simulink model "torqueBalancingSOT2012b"  (Simulink 8.0)
settings: Solver=FixedStepDiscrete  StartTime=0.0  StopTime=CONFIG.SIMULATION_TIME  FixedStep=CONFIG.Ts  RelTol=1e-3
InitFcn:
  | cd(fileparts(which(bdroot)));
  | initTorqueBalancingSOT;
undefined symbols (not defined in the file or in its folder): CONFIG, ConstraintsFeetMatrix, gain, ROBOT_DOF, sat, sm, upperBoundFeetConstraints, WBT_robotName
libraries: WBToolboxLibrary x51
(part 1 of 2)
settings Model: Creator=marie  LastModifiedBy=marie  CovMetricSettings=dwe  CovHtmlReporting=off  covSaveCumulativeToWorkspaceVar=off  CovSaveSingleToWorkspaceVar=off  CovExternalEMLEnable=on
settings DataIOCC: LimitDataPoints=off  SaveFormat=StructureWithTime
settings OptimizationCC: ExpressionDepthLimit=128
settings DebuggingCC: UnderspecifiedInitializationDetection=Simplified  MergeDetectMultiDrivingBlocksExec=error  SolverPrmCheckMsg=none  FrameProcessingCompatibilityMsg=error  StateNameClashWarn=none  SFUnexpectedBacktrackingDiag=error  SFNoUnconditionalDefaultTransitionDiag=error
settings HardwareCC: ProdBitPerPointer=64  ProdLargestAtomicFloat=Float  ProdIntDivRoundTo=Zero  ProdEndianess=LittleEndian  ProdHWDeviceType=Specified
settings ModelReferenceCC: PropagateSignalLabelsOutOfModel=on
settings CodeAppCC: CustomSymbolStrType=$N$R$M_T
settings GRTTargetCC: CodeReplacementLibrary=C99 (ISO)  GeneratePreprocessorConditionals=Use local settings

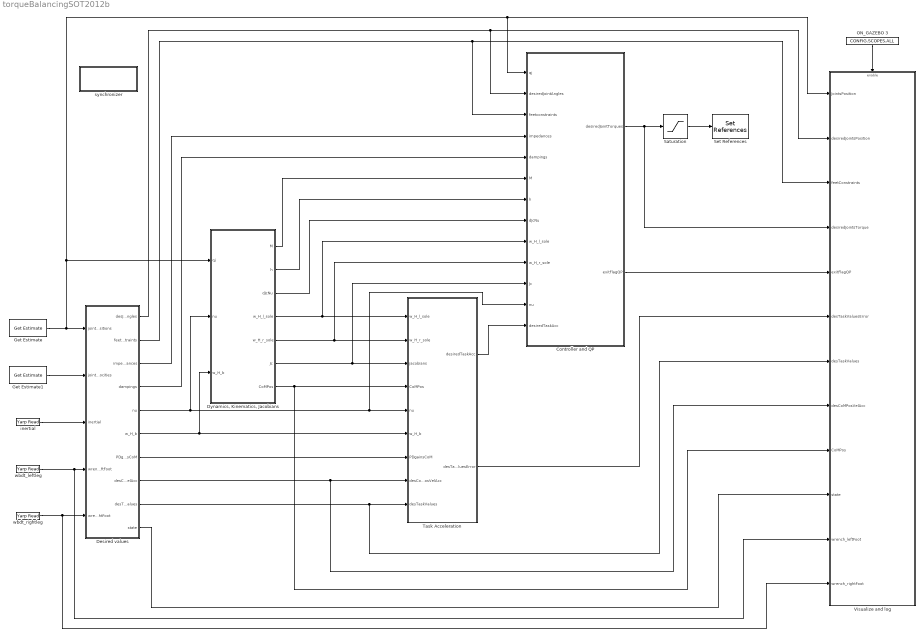
== system torqueBalancingSOT2012b ==
  Controller and QP : Subsystem
  Desired values : Subsystem
  "Dynamics, Kinematics, Jacobians" : Subsystem
  Get Estimate : WBToolboxLibrary/wholeBodyStates/Get Estimate  estimateType=Joints Position  robotName=WBT_robotName  localName=WBT_modelName  wbiFile=WBT_wbiFilename  wbiList=WBT_wbiList
  Get Estimate1 : WBToolboxLibrary/wholeBodyStates/Get Estimate  estimateType=Joints Velocity  robotName=WBT_robotName  localName=WBT_modelName  wbiFile=WBT_wbiFilename  wbiList=WBT_wbiList
  ON_GAZEBO 3 : Constant  Value=CONFIG.SCOPES.ALL
  Saturation : Saturate  UpperLimit=sat.torque  LowerLimit=-sat.torque
  Set References : WBToolboxLibrary/wholeBodyActuators/Set References  controlType=Torque  fullOrSubControl=Full  controlledJoints=''  robotName=WBT_robotName  localName=WBT_modelName  wbiFile=WBT_wbiFilename  wbiList=WBT_wbiList
  Task Acceleration : Subsystem
  Visualize and log : Subsystem
  inertial : WBToolboxLibrary/Utilities/Yarp Read  portName=PORTS.IMU  signalSize=12  blocking=off  timestamp=off  autoconnect=on  errorOnConnection=on
  synchronizer : Subsystem
      mask Display: disp('SYNCHRONIZER')
  wbdt_leftleg : WBToolboxLibrary/Utilities/Yarp Read  portName=PORTS.WBDT_LEFTLEG_EE  signalSize=6  blocking=off  timestamp=off  autoconnect=on  errorOnConnection=off
  wbdt_rightleg : WBToolboxLibrary/Utilities/Yarp Read  portName=PORTS.WBDT_RIGHTLEG_EE  signalSize=6  blocking=off  timestamp=off  autoconnect=on  errorOnConnection=off
  wires:
  Desired values/6(w_H_b) -> Task Acceleration/6(w_H_b), "Dynamics, Kinematics, Jacobians"/3(w_H_b)
  Get Estimate/1 -> "Dynamics, Kinematics, Jacobians"/1(qj), Visualize and log/1(JointsPosition), Controller and QP/1(qj), Desired values/1(jointPositions)
  "Dynamics, Kinematics, Jacobians"/7(CoMPos) -> Visualize and log/9(CoMPos), Task Acceleration/4(CoMPos)
  Desired values/8(desCoMPosVelAcc) -> Visualize and log/8(desCoMPosVelAcc), Task Acceleration/8(desCoMPosVelAcc)
  Desired values/5(nu) -> Controller and QP/12(nu), Task Acceleration/5(nu), "Dynamics, Kinematics, Jacobians"/2(nu)
  "Dynamics, Kinematics, Jacobians"/6(Jc) -> Controller and QP/11(Jc), Task Acceleration/3(jacobians)
  Desired values/1(desJointAngles) -> Controller and QP/2(desiredJointAngles), Visualize and log/2(desiredJointsPosition)
  Desired values/9(desTaskValues) -> Task Acceleration/9(desTaskValues), Visualize and log/7(desTaskValues)
  Desired values/7(PDgainsCoM) -> Task Acceleration/7(PDgainsCoM)
  "Dynamics, Kinematics, Jacobians"/5(w_H_r_sole) -> Controller and QP/10(w_H_r_sole), Task Acceleration/2(w_H_r_sole)
  "Dynamics, Kinematics, Jacobians"/4(w_H_l_sole) -> Controller and QP/9(w_H_l_sole), Task Acceleration/1(w_H_l_sole)
  Desired values/3(impedances) -> Controller and QP/4(impedances)
  Desired values/2(feetConstraints) -> Visualize and log/3(feetConstraints), Controller and QP/3(feetconstraints)
  "Dynamics, Kinematics, Jacobians"/1(M) -> Controller and QP/6(M)
  "Dynamics, Kinematics, Jacobians"/2(h) -> Controller and QP/7(h)
  "Dynamics, Kinematics, Jacobians"/3(dJcNu) -> Controller and QP/8(dJcNu)
  Task Acceleration/1(desiredTaskAcc) -> Controller and QP/13(desiredTaskAcc)
  Desired values/4(dampings) -> Controller and QP/5(dampings)
  Controller and QP/1(desiredJointTorques) -> Visualize and log/4(desiredJointsTorque), Saturation/1
  Saturation/1 -> Set References/1
  ON_GAZEBO 3/1 -> Visualize and log/Enable
  Desired values/10(state) -> Visualize and log/10(state)
  Controller and QP/2(exitFlagQP) -> Visualize and log/5(exitFlagQP)
  Task Acceleration/2(desTaskValuesError) -> Visualize and log/6(desTaskValuesError)
  inertial/1 -> Desired values/3(inertial)
  wbdt_leftleg/1 -> Desired values/4(wrench_leftFoot), Visualize and log/11(wrench_leftFoot)
  wbdt_rightleg/1 -> Desired values/5(wrench_rightFoot), Visualize and log/12(wrench_rightFoot)
  Get Estimate1/1 -> Desired values/2(jointVelocities)

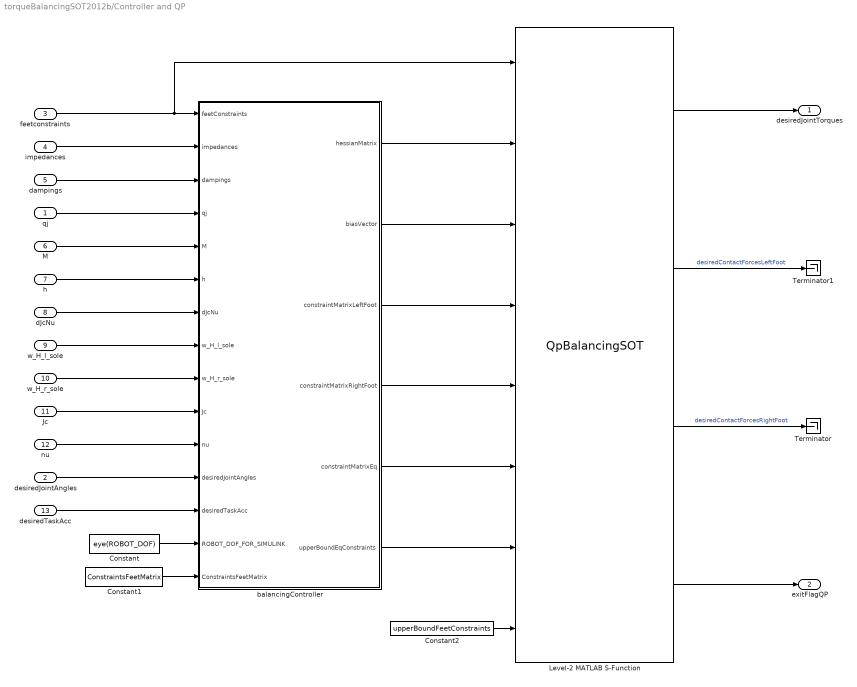
== system torqueBalancingSOT2012b/Controller and QP ==
  qj : Inport
  desiredJointAngles : Inport  Port=2
  feetconstraints : Inport  Port=3
  impedances : Inport  Port=4
  dampings : Inport  Port=5
  M : Inport  Port=6
  h : Inport  Port=7
  dJcNu : Inport  Port=8
  w_H_l_sole : Inport  Port=9
  w_H_r_sole : Inport  Port=10
  Jc : Inport  Port=11
  nu : Inport  Port=12
  desiredTaskAcc : Inport  Port=13
  Constant : Constant  Value=eye(ROBOT_DOF)
  Constant1 : Constant  Value=ConstraintsFeetMatrix
  Constant2 : Constant  Value=upperBoundFeetConstraints
  Level-2 MATLAB S-Function : M-S-Function  FunctionName=QpBalancingSOT  Parameters=ROBOT_DOF,sat.torqueDot,CONFIG.Ts,CONFIG.QP.USE_CONTINUITY_CONSTRAINTS,CONFIG.QP.USE_STRICT_TASK_PRIORITIES, reg.HessianQP  mask{robotDofs=ROBOT_DOF, tauDotMax=sat.torqueDot, Ts=CONFIG.Ts}
      mask prompts: robotDofs "Robt degrees of freedom"; tauDotMax "Maximum derivative of torques"; Ts "Controller period"
      mask Display: disp('QP')
  Terminator : Terminator
  Terminator1 : Terminator
  balancingController : MATLAB Function  TreatAsAtomicUnit=on
      settings: PermitHierarchicalResolution=ParametersOnly
  desiredJointTorques : Outport
  exitFlagQP : Outport  Port=2
  wires:
  balancingController/1(hessianMatrix) -> Level-2 MATLAB S-Function/2
  feetconstraints/1 -> balancingController/1(feetConstraints), Level-2 MATLAB S-Function/1
  qj/1 -> balancingController/4(qj)
  impedances/1 -> balancingController/2(impedances)
  M/1 -> balancingController/5(M)
  h/1 -> balancingController/6(h)
  dJcNu/1 -> balancingController/7(dJcNu)
  w_H_l_sole/1 -> balancingController/8(w_H_l_sole)
  w_H_r_sole/1 -> balancingController/9(w_H_r_sole)
  Jc/1 -> balancingController/10(Jc)
  nu/1 -> balancingController/11(nu)
  desiredJointAngles/1 -> balancingController/12(desiredJointAngles)
  desiredTaskAcc/1 -> balancingController/13(desiredTaskAcc)
  Constant/1 -> balancingController/14(ROBOT_DOF_FOR_SIMULINK)
  Constant1/1 -> balancingController/15(ConstraintsFeetMatrix)
  dampings/1 -> balancingController/3(dampings)
  balancingController/2(biasVector) -> Level-2 MATLAB S-Function/3
  balancingController/3(constraintMatrixLeftFoot) -> Level-2 MATLAB S-Function/4
  balancingController/4(constraintMatrixRightFoot) -> Level-2 MATLAB S-Function/5
  balancingController/5(constraintMatrixEq) -> Level-2 MATLAB S-Function/6
  balancingController/6(upperBoundEqConstraints) -> Level-2 MATLAB S-Function/7
  Constant2/1 -> Level-2 MATLAB S-Function/8
  Level-2 MATLAB S-Function/1 -> desiredJointTorques/1
  Level-2 MATLAB S-Function/2 -> Terminator1/1  "desiredContactForcesLeftFoot"
  Level-2 MATLAB S-Function/3 -> Terminator/1  "desiredContactForcesRightFoot"
  Level-2 MATLAB S-Function/4 -> exitFlagQP/1

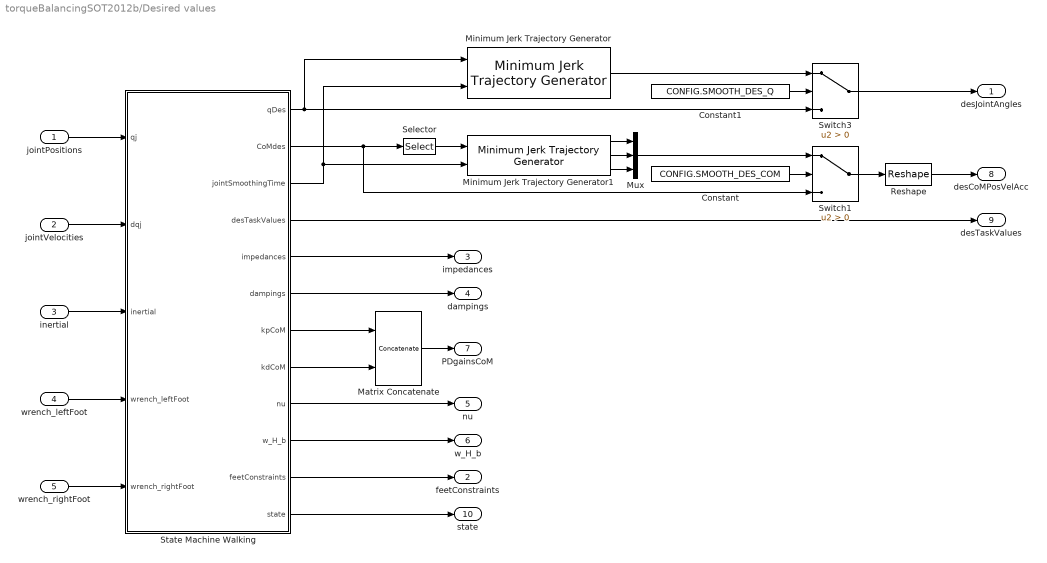
== system torqueBalancingSOT2012b/Desired values ==
  jointPositions : Inport
  jointVelocities : Inport  Port=2
  inertial : Inport  Port=3
  wrench_leftFoot : Inport  Port=4
  wrench_rightFoot : Inport  Port=5
  Constant : Constant  Value=CONFIG.SMOOTH_DES_COM
  Constant1 : Constant  Value=CONFIG.SMOOTH_DES_Q
  Matrix Concatenate : Concatenate  Mode=Multidimensional array  ConcatenateDimension=2
  Minimum Jerk Trajectory Generator : WBToolboxLibrary/Utilities/Minimum Jerk Trajectory Generator  externalSettlingTime=on  settlingTime=3  sampleTime=CONFIG.Ts  resetOnSettlingTime=off  firstDerivatives=off  secondDerivatives=off  explicitInitialValue=off
  Minimum Jerk Trajectory Generator1 : WBToolboxLibrary/Utilities/Minimum Jerk Trajectory Generator  externalSettlingTime=on  settlingTime=3  sampleTime=CONFIG.Ts  resetOnSettlingTime=off  firstDerivatives=on  secondDerivatives=on  explicitInitialValue=off
  Mux : Mux  Inputs=3
  Reshape : Reshape  OutputDimensionality=Customize  OutputDimensions=[3,3]
  Selector : Selector  InputPortWidth=9  IndexOptions=Index vector (dialog)  Indices=[1 2 3]  OutputSizes=1
  State Machine Walking : Subsystem
  Switch1 : Switch  Criteria=u2 > Threshold
  Switch3 : Switch  Criteria=u2 > Threshold
  desJointAngles : Outport
  feetConstraints : Outport  Port=2
  impedances : Outport  Port=3
  dampings : Outport  Port=4
  nu : Outport  Port=5
  w_H_b : Outport  Port=6
  PDgainsCoM : Outport  Port=7
  desCoMPosVelAcc : Outport  Port=8
  desTaskValues : Outport  Port=9
  state : Outport  Port=10
  wires:
  Minimum Jerk Trajectory Generator/1 -> Switch3/1
  Constant/1 -> Switch1/2
  Constant1/1 -> Switch3/2
  Minimum Jerk Trajectory Generator1/3 -> Mux/3
  Minimum Jerk Trajectory Generator1/2 -> Mux/2
  State Machine Walking/8(kdCoM) -> Matrix Concatenate/2
  Matrix Concatenate/1 -> PDgainsCoM/1
  State Machine Walking/10(w_H_b) -> w_H_b/1
  State Machine Walking/12(state) -> state/1
  Mux/1 -> Switch1/1
  Minimum Jerk Trajectory Generator1/1 -> Mux/1
  State Machine Walking/5(impedances) -> impedances/1
  Selector/1 -> Minimum Jerk Trajectory Generator1/1
  State Machine Walking/3(jointSmoothingTime) -> Minimum Jerk Trajectory Generator/2, Minimum Jerk Trajectory Generator1/2
  Switch1/1 -> Reshape/1
  Switch3/1 -> desJointAngles/1
  State Machine Walking/2(CoMdes) -> Switch1/3, Selector/1
  State Machine Walking/4(desTaskValues) -> desTaskValues/1
  State Machine Walking/11(feetConstraints) -> feetConstraints/1
  State Machine Walking/1(qDes) -> Minimum Jerk Trajectory Generator/1, Switch3/3
  State Machine Walking/9(nu) -> nu/1
  State Machine Walking/7(kpCoM) -> Matrix Concatenate/1
  Reshape/1 -> desCoMPosVelAcc/1
  jointPositions/1 -> State Machine Walking/1(qj)
  jointVelocities/1 -> State Machine Walking/2(dqj)
  State Machine Walking/6(dampings) -> dampings/1
  wrench_rightFoot/1 -> State Machine Walking/5(wrench_rightFoot)
  wrench_leftFoot/1 -> State Machine Walking/4(wrench_leftFoot)
  inertial/1 -> State Machine Walking/3(inertial)

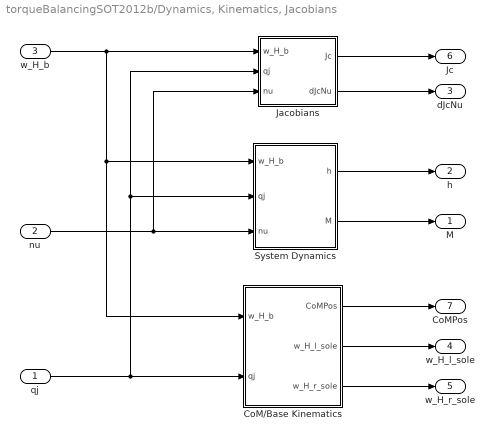
== system torqueBalancingSOT2012b/Dynamics, Kinematics, Jacobians ==
  qj : Inport
  nu : Inport  Port=2
  w_H_b : Inport  Port=3
  CoM/Base Kinematics : Subsystem
  Jacobians : Subsystem
  System Dynamics : Subsystem
  M : Outport
  h : Outport  Port=2
  dJcNu : Outport  Port=3
  w_H_l_sole : Outport  Port=4
  w_H_r_sole : Outport  Port=5
  Jc : Outport  Port=6
  CoMPos : Outport  Port=7
  wires:
  qj/1 -> Jacobians/2(qj), System Dynamics/2(qj), CoM/Base Kinematics/2(qj)
  w_H_b/1 -> CoM/Base Kinematics/1(w_H_b), System Dynamics/1(w_H_b), Jacobians/1(w_H_b)
  CoM/Base Kinematics/1(CoMPos) -> CoMPos/1
  nu/1 -> Jacobians/3(nu), System Dynamics/3(nu)
  Jacobians/1(Jc) -> Jc/1
  Jacobians/2(dJcNu) -> dJcNu/1
  System Dynamics/2(M) -> M/1
  System Dynamics/1(h) -> h/1
  CoM/Base Kinematics/2(w_H_l_sole) -> w_H_l_sole/1
  CoM/Base Kinematics/3(w_H_r_sole) -> w_H_r_sole/1

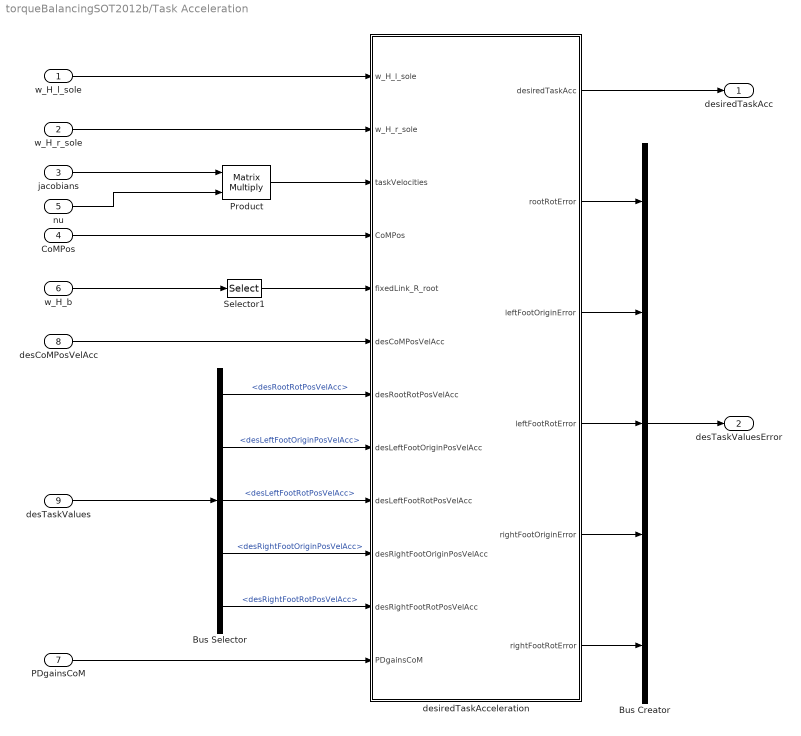
== system torqueBalancingSOT2012b/Task Acceleration ==
  w_H_l_sole : Inport
  w_H_r_sole : Inport  Port=2
  jacobians : Inport  Port=3
  CoMPos : Inport  Port=4
  nu : Inport  Port=5
  w_H_b : Inport  Port=6
  PDgainsCoM : Inport  Port=7
  desCoMPosVelAcc : Inport  Port=8
  desTaskValues : Inport  Port=9
  Bus Creator : BusCreator  Inputs='rootRotError','leftFootOriginError','leftFootRotError','rightFootOriginError','rightFootRotError'
  Bus Selector : BusSelector  OutputSignals=desRootRotPosVelAcc,desLeftFootOriginPosVelAcc,desLeftFootRotPosVelAcc,desRightFootOriginPosVelAcc,desRightFootRotPosVelAcc
  Product : Product  Multiplication=Matrix(*)
  Selector1 : Selector  NumberOfDimensions=2  InputPortWidth=9  IndexOptions=Index vector (dialog),Index vector (dialog)  Indices=[1:3],[1:3]  OutputSizes=1,1
  desiredTaskAcceleration : MATLAB Function  TreatAsAtomicUnit=on
      settings: PermitHierarchicalResolution=ParametersOnly
  desiredTaskAcc : Outport
  desTaskValuesError : Outport  Port=2
  wires:
  Bus Selector/1 -> desiredTaskAcceleration/7(desRootRotPosVelAcc)  "<desRootRotPosVelAcc>"
  Bus Selector/2 -> desiredTaskAcceleration/8(desLeftFootOriginPosVelAcc)  "<desLeftFootOriginPosVelAcc>"
  Bus Selector/3 -> desiredTaskAcceleration/9(desLeftFootRotPosVelAcc)  "<desLeftFootRotPosVelAcc>"
  Bus Selector/4 -> desiredTaskAcceleration/10(desRightFootOriginPosVelAcc)  "<desRightFootOriginPosVelAcc>"
  desTaskValues/1 -> Bus Selector/1
  w_H_b/1 -> Selector1/1
  Bus Selector/5 -> desiredTaskAcceleration/11(desRightFootRotPosVelAcc)  "<desRightFootRotPosVelAcc>"
  PDgainsCoM/1 -> desiredTaskAcceleration/12(PDgainsCoM)
  jacobians/1 -> Product/1
  nu/1 -> Product/2
  CoMPos/1 -> desiredTaskAcceleration/4(CoMPos)
  desCoMPosVelAcc/1 -> desiredTaskAcceleration/6(desCoMPosVelAcc)
  Product/1 -> desiredTaskAcceleration/3(taskVelocities)
  desiredTaskAcceleration/2(rootRotError) -> Bus Creator/1
  desiredTaskAcceleration/3(leftFootOriginError) -> Bus Creator/2
  desiredTaskAcceleration/4(leftFootRotError) -> Bus Creator/3
  desiredTaskAcceleration/5(rightFootOriginError) -> Bus Creator/4
  desiredTaskAcceleration/6(rightFootRotError) -> Bus Creator/5
  desiredTaskAcceleration/1(desiredTaskAcc) -> desiredTaskAcc/1
  Bus Creator/1 -> desTaskValuesError/1
  w_H_r_sole/1 -> desiredTaskAcceleration/2(w_H_r_sole)
  w_H_l_sole/1 -> desiredTaskAcceleration/1(w_H_l_sole)
  Selector1/1 -> desiredTaskAcceleration/5(fixedLink_R_root)

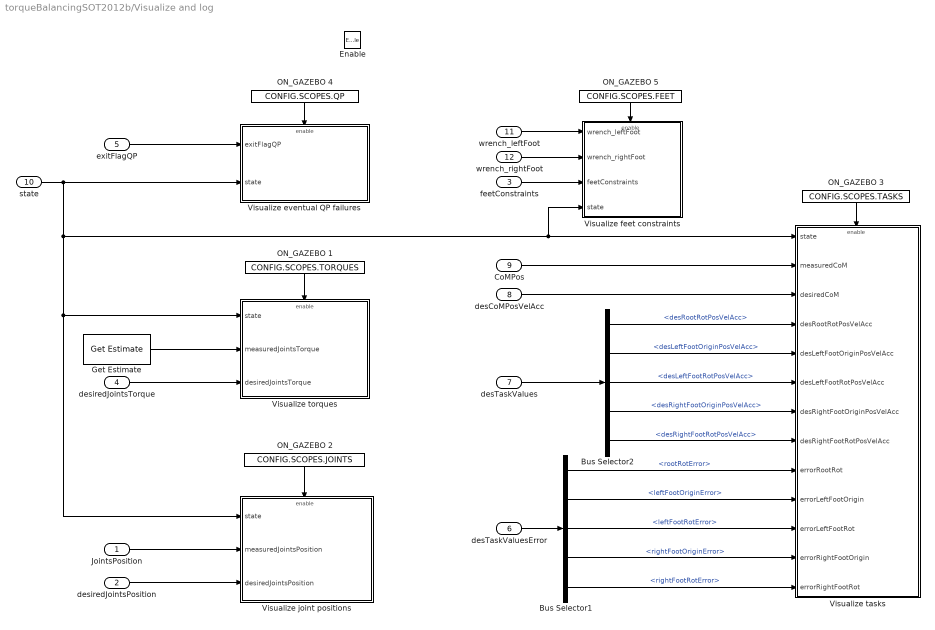
== system torqueBalancingSOT2012b/Visualize and log ==
  JointsPosition : Inport
  desiredJointsPosition : Inport  Port=2
  feetConstraints : Inport  Port=3
  desiredJointsTorque : Inport  Port=4
  exitFlagQP : Inport  Port=5
  desTaskValuesError : Inport  Port=6
  desTaskValues : Inport  Port=7
  desCoMPosVelAcc : Inport  Port=8
  CoMPos : Inport  Port=9
  state : Inport  Port=10
  wrench_leftFoot : Inport  Port=11
  wrench_rightFoot : Inport  Port=12
  Enable : EnablePort
  Bus Selector1 : BusSelector  OutputSignals=rootRotError,leftFootOriginError,leftFootRotError,rightFootOriginError,rightFootRotError
  Bus Selector2 : BusSelector  OutputSignals=desRootRotPosVelAcc,desLeftFootOriginPosVelAcc,desLeftFootRotPosVelAcc,desRightFootOriginPosVelAcc,desRightFootRotPosVelAcc
  Get Estimate : WBToolboxLibrary/wholeBodyStates/Get Estimate  estimateType=Joints Torque  robotName=WBT_robotName  localName=WBT_modelName  wbiFile=WBT_wbiFilename  wbiList=WBT_wbiList
  ON_GAZEBO 1 : Constant  Value=CONFIG.SCOPES.TORQUES
  ON_GAZEBO 2 : Constant  Value=CONFIG.SCOPES.JOINTS
  ON_GAZEBO 3 : Constant  Value=CONFIG.SCOPES.TASKS
  ON_GAZEBO 4 : Constant  Value=CONFIG.SCOPES.QP
  ON_GAZEBO 5 : Constant  Value=CONFIG.SCOPES.FEET
  Visualize eventual QP failures : Subsystem
  Visualize feet constraints : Subsystem
  Visualize joint positions : Subsystem
  Visualize tasks : Subsystem
  Visualize torques : Subsystem
  wires:
  ON_GAZEBO 4/1 -> Visualize eventual QP failures/Enable
  exitFlagQP/1 -> Visualize eventual QP failures/1(exitFlagQP)
  Get Estimate/1 -> Visualize torques/2(measuredJointsTorque)
  desiredJointsTorque/1 -> Visualize torques/3(desiredJointsTorque)
  ON_GAZEBO 1/1 -> Visualize torques/Enable
  state/1 -> Visualize eventual QP failures/2(state), Visualize joint positions/1(state), Visualize torques/1(state), Visualize feet constraints/4(state), Visualize tasks/1(state)
  JointsPosition/1 -> Visualize joint positions/2(measuredJointsPosition)
  desiredJointsPosition/1 -> Visualize joint positions/3(desiredJointsPosition)
  ON_GAZEBO 2/1 -> Visualize joint positions/Enable
  CoMPos/1 -> Visualize tasks/2(measuredCoM)
  desCoMPosVelAcc/1 -> Visualize tasks/3(desiredCoM)
  Bus Selector2/3 -> Visualize tasks/6(desLeftFootRotPosVelAcc)  "<desLeftFootRotPosVelAcc>"
  Bus Selector2/2 -> Visualize tasks/5(desLeftFootOriginPosVelAcc)  "<desLeftFootOriginPosVelAcc>"
  Bus Selector2/5 -> Visualize tasks/8(desRightFootRotPosVelAcc)  "<desRightFootRotPosVelAcc>"
  Bus Selector2/4 -> Visualize tasks/7(desRightFootOriginPosVelAcc)  "<desRightFootOriginPosVelAcc>"
  desTaskValues/1 -> Bus Selector2/1
  Bus Selector2/1 -> Visualize tasks/4(desRootRotPosVelAcc)  "<desRootRotPosVelAcc>"
  desTaskValuesError/1 -> Bus Selector1/1
  Bus Selector1/1 -> Visualize tasks/9(errorRootRot)  "<rootRotError>"
  Bus Selector1/2 -> Visualize tasks/10(errorLeftFootOrigin)  "<leftFootOriginError>"
  Bus Selector1/3 -> Visualize tasks/11(errorLeftFootRot)  "<leftFootRotError>"
  Bus Selector1/4 -> Visualize tasks/12(errorRightFootOrigin)  "<rightFootOriginError>"
  Bus Selector1/5 -> Visualize tasks/13(errorRightFootRot)  "<rightFootRotError>"
  ON_GAZEBO 3/1 -> Visualize tasks/Enable
  feetConstraints/1 -> Visualize feet constraints/3(feetConstraints)
  ON_GAZEBO 5/1 -> Visualize feet constraints/Enable
  wrench_rightFoot/1 -> Visualize feet constraints/2(wrench_rightFoot)
  wrench_leftFoot/1 -> Visualize feet constraints/1(wrench_leftFoot)

== system torqueBalancingSOT2012b/synchronizer ==
  GAZEBO_SYNCHRONIZER : Subsystem
  Logical Operator : Logic  Operator=NOT  AllPortsSameDT=off  OutDataTypeStr=boolean
  "ON_GAZEBO " : Constant  Value=CONFIG.ON_GAZEBO
  REAL_TIME_SYNC : Subsystem
  wires:
  Logical Operator/1 -> REAL_TIME_SYNC/Enable
  "ON_GAZEBO "/1 -> GAZEBO_SYNCHRONIZER/Enable, Logical Operator/1

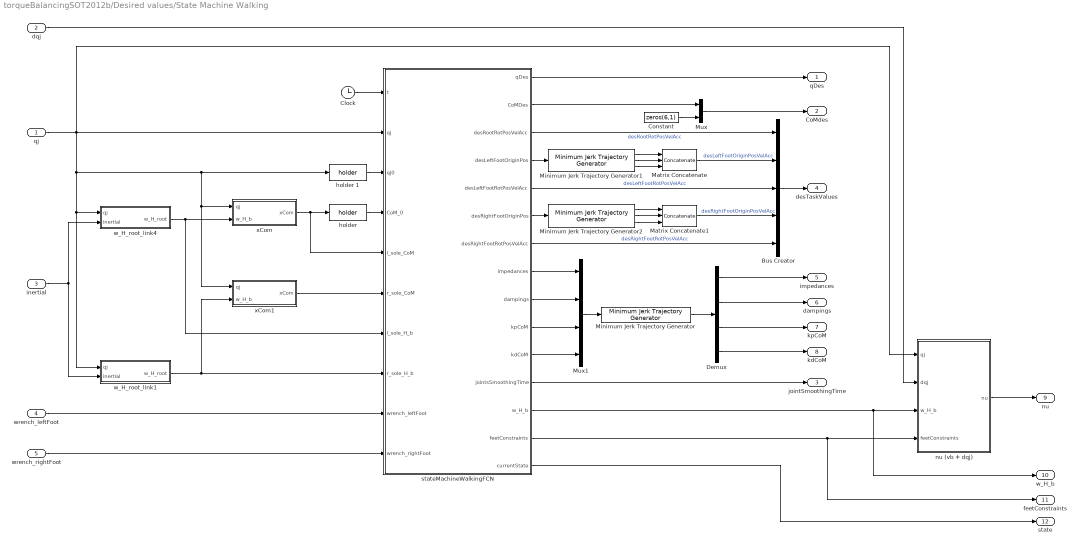
== system torqueBalancingSOT2012b/Desired values/State Machine Walking ==
  qj : Inport
  dqj : Inport  Port=2
  inertial : Inport  Port=3
  wrench_leftFoot : Inport  Port=4
  wrench_rightFoot : Inport  Port=5
  Bus Creator : BusCreator  Inputs='desRootRotPosVelAcc','desLeftFootOriginPosVelAcc','desLeftFootRotPosVelAcc','desRightFootOriginPosVelAcc','desRightFootRotPosVelAcc'
  Clock : Clock
  Constant : Constant  Value=zeros(6,1)
  Demux : Demux  Outputs=[ROBOT_DOF, ROBOT_DOF, 3, 3]
  Matrix Concatenate : Concatenate  NumInputs=3  Mode=Multidimensional array  ConcatenateDimension=2
  Matrix Concatenate1 : Concatenate  NumInputs=3  Mode=Multidimensional array  ConcatenateDimension=2
  Minimum Jerk Trajectory Generator : WBToolboxLibrary/Utilities/Minimum Jerk Trajectory Generator  externalSettlingTime=off  settlingTime=gain.SmoothingTimeGainScheduling  sampleTime=CONFIG.Ts  resetOnSettlingTime=off  firstDerivatives=off  secondDerivatives=off  explicitInitialValue=off
  Minimum Jerk Trajectory Generator1 : WBToolboxLibrary/Utilities/Minimum Jerk Trajectory Generator  externalSettlingTime=off  settlingTime=gain.SmoothingTimeGainScheduling  sampleTime=CONFIG.Ts  resetOnSettlingTime=off  firstDerivatives=on  secondDerivatives=on  explicitInitialValue=off
  Minimum Jerk Trajectory Generator2 : WBToolboxLibrary/Utilities/Minimum Jerk Trajectory Generator  externalSettlingTime=off  settlingTime=gain.SmoothingTimeGainScheduling  sampleTime=CONFIG.Ts  resetOnSettlingTime=off  firstDerivatives=on  secondDerivatives=on  explicitInitialValue=off
  Mux : Mux  Inputs=2
  Mux1 : Mux
  "holder " : WBToolboxLibrary/Utilities/holder 
  holder 1 : WBToolboxLibrary/Utilities/holder 
  nu (vb + dqj) : Subsystem
  stateMachineWalkingFCN : MATLAB Function  TreatAsAtomicUnit=on
      settings: PermitHierarchicalResolution=ParametersOnly
  w_H_root_link1 : Subsystem  mask{link_name='r_sole'}
      mask prompts: link_name "link name"
      mask help:
      | This block evaluates the homogeneous transformation between the world and the root link, i.e. ^wH_b. It assumes that the link specified by the variable 'link_name' has a constant position
      | w.r.t. an inertial frame, but it can rotate arbitrarily. This rotation is retrived from the IMU sensor.
      mask Display:
      | str = strrep(link_name, '_','\_');
      | port_label('output',1,['{}^{',str '}H_{root}'],'texmode','on')
      | clear str;
      | 
      | port_label('input',1,'q_j','texmode','on')
      | 
      | port_label('input',2,'inertial','texmode','on')
  w_H_root_link4 : Subsystem  mask{link_name='l_sole'}
      mask prompts: link_name "link name"
      mask help:
      | This block evaluates the homogeneous transformation between the world and the root link, i.e. ^wH_b. It assumes that the link specified by the variable 'link_name' has a constant position
      | w.r.t. an inertial frame, but it can rotate arbitrarily. This rotation is retrived from the IMU sensor.
      mask Display:
      | str = strrep(link_name, '_','\_');
      | port_label('output',1,['{}^{',str '}H_{root}'],'texmode','on')
      | clear str;
      | 
      | port_label('input',1,'q_j','texmode','on')
      | 
      | port_label('input',2,'inertial','texmode','on')
  xCom : Subsystem
  xCom1 : Subsystem
  qDes : Outport
  CoMdes : Outport  Port=2
  jointSmoothingTime : Outport  Port=3
  desTaskValues : Outport  Port=4
  impedances : Outport  Port=5
  dampings : Outport  Port=6
  kpCoM : Outport  Port=7
  kdCoM : Outport  Port=8
  nu : Outport  Port=9
  w_H_b : Outport  Port=10
  feetConstraints : Outport  Port=11
  state : Outport  Port=12
  wires:
  Clock/1 -> stateMachineWalkingFCN/1(t)
  stateMachineWalkingFCN/8(impedances) -> Mux1/1
  stateMachineWalkingFCN/11(kdCoM) -> Mux1/4
  stateMachineWalkingFCN/7(desRightFootRotPosVelAcc) -> Bus Creator/5  "desRightFootRotPosVelAcc"
  Bus Creator/1 -> desTaskValues/1
  wrench_rightFoot/1 -> stateMachineWalkingFCN/10(wrench_rightFoot)
  stateMachineWalkingFCN/10(kpCoM) -> Mux1/3
  stateMachineWalkingFCN/13(w_H_b) -> w_H_b/1, nu (vb + dqj)/3(w_H_b)
  wrench_leftFoot/1 -> stateMachineWalkingFCN/9(wrench_leftFoot)
  Mux1/1 -> Minimum Jerk Trajectory Generator/1
  qj/1 -> nu (vb + dqj)/1(qj), w_H_root_link1/1(qj), w_H_root_link4/1(qj), xCom1/1(qj), xCom/1(qj), holder 1/1, stateMachineWalkingFCN/2(qj)
  nu (vb + dqj)/1(nu) -> nu/1
  holder 1/1 -> stateMachineWalkingFCN/3(qj0)
  xCom1/1(xCom) -> stateMachineWalkingFCN/6(r_sole_CoM)
  "holder "/1 -> stateMachineWalkingFCN/4(CoM_0)
  w_H_root_link4/1(w_H_root) -> stateMachineWalkingFCN/7(l_sole_H_b), xCom/2(w_H_b)
  inertial/1 -> w_H_root_link4/2(inertial), w_H_root_link1/2(inertial)
  xCom/1(xCom) -> "holder "/1, stateMachineWalkingFCN/5(l_sole_CoM)
  Minimum Jerk Trajectory Generator/1 -> Demux/1
  stateMachineWalkingFCN/14(feetConstraints) -> nu (vb + dqj)/4(feetConstraints), feetConstraints/1
  dqj/1 -> nu (vb + dqj)/2(dqj)
  stateMachineWalkingFCN/2(CoMDes) -> Mux/1
  w_H_root_link1/1(w_H_root) -> stateMachineWalkingFCN/8(r_sole_H_b), xCom1/2(w_H_b)
  Demux/1 -> impedances/1
  stateMachineWalkingFCN/12(jointsSmoothingTime) -> jointSmoothingTime/1
  stateMachineWalkingFCN/15(currentState) -> state/1
  stateMachineWalkingFCN/1(qDes) -> qDes/1
  Demux/3 -> kpCoM/1
  Minimum Jerk Trajectory Generator1/1 -> Matrix Concatenate/1
  Minimum Jerk Trajectory Generator1/2 -> Matrix Concatenate/2
  Minimum Jerk Trajectory Generator1/3 -> Matrix Concatenate/3
  Matrix Concatenate/1 -> Bus Creator/2  "desLeftFootOriginPosVelAcc"
  stateMachineWalkingFCN/4(desLeftFootOriginPos) -> Minimum Jerk Trajectory Generator1/1
  Minimum Jerk Trajectory Generator2/1 -> Matrix Concatenate1/1
  Minimum Jerk Trajectory Generator2/2 -> Matrix Concatenate1/2
  Minimum Jerk Trajectory Generator2/3 -> Matrix Concatenate1/3
  stateMachineWalkingFCN/6(desRightFootOriginPos) -> Minimum Jerk Trajectory Generator2/1
  Matrix Concatenate1/1 -> Bus Creator/4  "desRightFootOriginPosVelAcc"
  stateMachineWalkingFCN/3(desRootRotPosVelAcc) -> Bus Creator/1  "desRootRotPosVelAcc"
  stateMachineWalkingFCN/5(desLeftFootRotPosVelAcc) -> Bus Creator/3  "desLeftFootRotPosVelAcc"
  Demux/4 -> kdCoM/1
  Constant/1 -> Mux/2
  Mux/1 -> CoMdes/1
  stateMachineWalkingFCN/9(dampings) -> Mux1/2
  Demux/2 -> dampings/1

== system torqueBalancingSOT2012b/Dynamics, Kinematics, Jacobians/CoM/Base Kinematics ==
  w_H_b : Inport
  qj : Inport  Port=2
  Forward Kinematics : WBToolboxLibrary/wholeBodyModel/Kinematics/Forward Kinematics  frameName='com'  robotName=WBT_robotName  localName=WBT_modelName  wbiFile=WBT_wbiFilename  wbiList=WBT_wbiList
  Forward Kinematics1 : WBToolboxLibrary/wholeBodyModel/Kinematics/Forward Kinematics  frameName='l_sole'  robotName=WBT_robotName  localName=WBT_modelName  wbiFile=WBT_wbiFilename  wbiList=WBT_wbiList
  Forward Kinematics2 : WBToolboxLibrary/wholeBodyModel/Kinematics/Forward Kinematics  frameName='r_sole'  robotName=WBT_robotName  localName=WBT_modelName  wbiFile=WBT_wbiFilename  wbiList=WBT_wbiList
  Selector : Selector  NumberOfDimensions=2  InputPortWidth=6+ROBOT_DOF  IndexOptions=Index vector (dialog),Index vector (dialog)  Indices=[1:3],[4]  OutputSizes=1,1
  CoMPos : Outport
  w_H_l_sole : Outport  Port=2
  w_H_r_sole : Outport  Port=3
  wires:
  Selector/1 -> CoMPos/1
  qj/1 -> Forward Kinematics1/2, Forward Kinematics2/2, Forward Kinematics/2
  Forward Kinematics/1 -> Selector/1
  w_H_b/1 -> Forward Kinematics1/1, Forward Kinematics2/1, Forward Kinematics/1
  Forward Kinematics2/1 -> w_H_r_sole/1
  Forward Kinematics1/1 -> w_H_l_sole/1

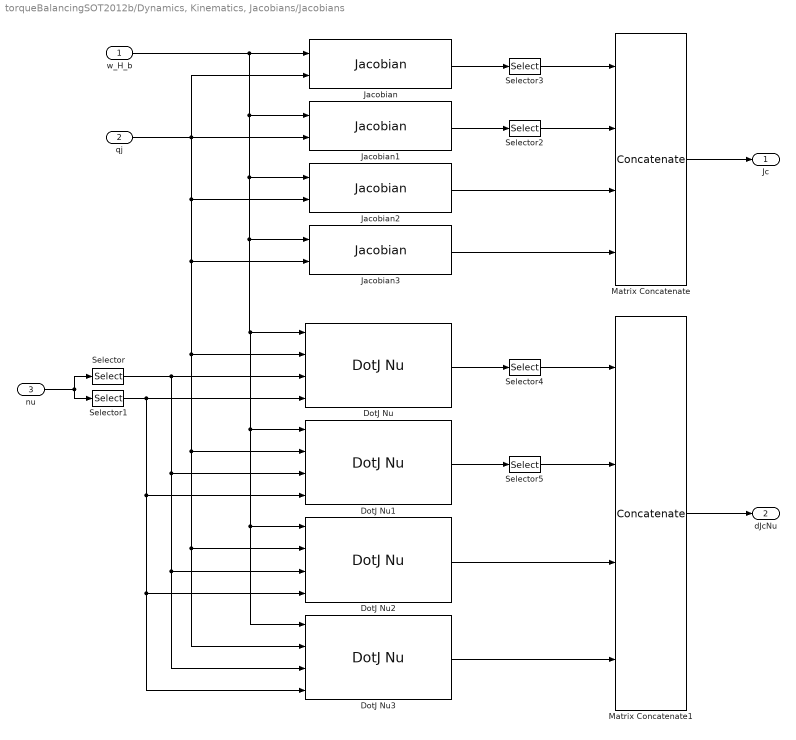
== system torqueBalancingSOT2012b/Dynamics, Kinematics, Jacobians/Jacobians ==
  w_H_b : Inport
  qj : Inport  Port=2
  nu : Inport  Port=3
  DotJ Nu : WBToolboxLibrary/wholeBodyModel/Jacobians/DotJ Nu  frameName='com'  robotName=WBT_robotName  localName=WBT_modelName  wbiFile=WBT_wbiFilename  wbiList=WBT_wbiList
  DotJ Nu1 : WBToolboxLibrary/wholeBodyModel/Jacobians/DotJ Nu  frameName='root_link'  robotName=WBT_robotName  localName=WBT_modelName  wbiFile=WBT_wbiFilename  wbiList=WBT_wbiList
  DotJ Nu2 : WBToolboxLibrary/wholeBodyModel/Jacobians/DotJ Nu  frameName='l_sole'  robotName=WBT_robotName  localName=WBT_modelName  wbiFile=WBT_wbiFilename  wbiList=WBT_wbiList
  DotJ Nu3 : WBToolboxLibrary/wholeBodyModel/Jacobians/DotJ Nu  frameName='r_sole'  robotName=WBT_robotName  localName=WBT_modelName  wbiFile=WBT_wbiFilename  wbiList=WBT_wbiList
  Jacobian : WBToolboxLibrary/wholeBodyModel/Jacobians/Jacobian  frameName='com'  robotName=WBT_robotName  localName=WBT_modelName  wbiFile=WBT_wbiFilename  wbiList=WBT_wbiList
  Jacobian1 : WBToolboxLibrary/wholeBodyModel/Jacobians/Jacobian  frameName='root_link'  robotName=WBT_robotName  localName=WBT_modelName  wbiFile=WBT_wbiFilename  wbiList=WBT_wbiList
  Jacobian2 : WBToolboxLibrary/wholeBodyModel/Jacobians/Jacobian  frameName='l_sole'  robotName=WBT_robotName  localName=WBT_modelName  wbiFile=WBT_wbiFilename  wbiList=WBT_wbiList
  Jacobian3 : WBToolboxLibrary/wholeBodyModel/Jacobians/Jacobian  frameName='r_sole'  robotName=WBT_robotName  localName=WBT_modelName  wbiFile=WBT_wbiFilename  wbiList=WBT_wbiList
  Matrix Concatenate : Concatenate  NumInputs=4  Mode=Multidimensional array
  Matrix Concatenate1 : Concatenate  NumInputs=4  Mode=Multidimensional array
  Selector : Selector  InputPortWidth=6+ROBOT_DOF  IndexOptions=Index vector (dialog)  Indices=[1:6]  OutputSizes=1
  Selector1 : Selector  InputPortWidth=6+ROBOT_DOF  IndexOptions=Index vector (dialog)  Indices=[7:6+ROBOT_DOF]  OutputSizes=1
  Selector2 : Selector  NumberOfDimensions=2  InputPortWidth=6+ROBOT_DOF  IndexOptions=Index vector (dialog),Index vector (dialog)  Indices=[4:6],[1:6+ROBOT_DOF]  OutputSizes=1,1
  Selector3 : Selector  NumberOfDimensions=2  InputPortWidth=6+ROBOT_DOF  IndexOptions=Index vector (dialog),Index vector (dialog)  Indices=[1:3],[1:6+ROBOT_DOF]  OutputSizes=1,1
  Selector4 : Selector  InputPortWidth=6  IndexOptions=Index vector (dialog)  Indices=[1:3]  OutputSizes=1
  Selector5 : Selector  InputPortWidth=6  IndexOptions=Index vector (dialog)  Indices=[4:6]  OutputSizes=1
  Jc : Outport
  dJcNu : Outport  Port=2
  wires:
  w_H_b/1 -> DotJ Nu1/1, DotJ Nu3/1, DotJ Nu2/1, DotJ Nu/1, Jacobian3/1, Jacobian2/1, Jacobian1/1, Jacobian/1
  qj/1 -> DotJ Nu3/2, DotJ Nu2/2, DotJ Nu1/2, DotJ Nu/2, Jacobian3/2, Jacobian2/2, Jacobian/2, Jacobian1/2
  Selector/1 -> DotJ Nu3/3, DotJ Nu2/3, DotJ Nu1/3, DotJ Nu/3
  Selector1/1 -> DotJ Nu1/4, DotJ Nu2/4, DotJ Nu3/4, DotJ Nu/4
  nu/1 -> Selector1/1, Selector/1
  Jacobian/1 -> Selector3/1
  Jacobian1/1 -> Selector2/1
  Selector3/1 -> Matrix Concatenate/1
  Selector2/1 -> Matrix Concatenate/2
  Jacobian2/1 -> Matrix Concatenate/3
  Jacobian3/1 -> Matrix Concatenate/4
  Matrix Concatenate/1 -> Jc/1
  DotJ Nu/1 -> Selector4/1
  DotJ Nu1/1 -> Selector5/1
  Selector4/1 -> Matrix Concatenate1/1
  Selector5/1 -> Matrix Concatenate1/2
  DotJ Nu2/1 -> Matrix Concatenate1/3
  DotJ Nu3/1 -> Matrix Concatenate1/4
  Matrix Concatenate1/1 -> dJcNu/1

== system torqueBalancingSOT2012b/Dynamics, Kinematics, Jacobians/System Dynamics ==
  w_H_b : Inport
  qj : Inport  Port=2
  nu : Inport  Port=3
  Get Bias Forces : WBToolboxLibrary/wholeBodyModel/Dynamics/Get Bias Forces  robotName=WBT_robotName  localName=WBT_modelName  wbiFile=WBT_wbiFilename  wbiList=WBT_wbiList  explicitGravity=off
  Mass Matrix : WBToolboxLibrary/wholeBodyModel/Dynamics/Mass Matrix  robotName=WBT_robotName  localName=WBT_modelName  wbiFile=WBT_wbiFilename  wbiList=WBT_wbiList
  Selector : Selector  InputPortWidth=6+ROBOT_DOF  IndexOptions=Index vector (dialog)  Indices=[1:6]  OutputSizes=1
  Selector1 : Selector  InputPortWidth=6+ROBOT_DOF  IndexOptions=Index vector (dialog)  Indices=[7:6+ROBOT_DOF]  OutputSizes=1
  h : Outport
  M : Outport  Port=2
  wires:
  Selector/1 -> Get Bias Forces/3
  Selector1/1 -> Get Bias Forces/4
  w_H_b/1 -> Get Bias Forces/1, Mass Matrix/1
  Get Bias Forces/1 -> h/1
  Mass Matrix/1 -> M/1
  qj/1 -> Get Bias Forces/2, Mass Matrix/2
  nu/1 -> Selector1/1, Selector/1

== system torqueBalancingSOT2012b/Visualize and log/Visualize eventual QP failures ==
  exitFlagQP : Inport
  state : Inport  Port=2
  Enable : EnablePort
  "QP status (0: no failure,  1: not using,  -1 internal error,  -2:  infeasible, -3:  unbounded) " : Scope  NumInputPorts=2
      settings: TimeRange=auto  ShowLegends=on  MaxDataPoints=5000  SaveToWorkspace=off  YMin=-1.00000~-0.25  YMax=1.00000~12.25  SampleTime=-1
  wires:
  exitFlagQP/1 -> "QP status (0: no failure,  1: not using,  -1 internal error,  -2:  infeasible, -3:  unbounded) "/1  "exitFlagQP"
  state/1 -> "QP status (0: no failure,  1: not using,  -1 internal error,  -2:  infeasible, -3:  unbounded) "/2

== system torqueBalancingSOT2012b/Visualize and log/Visualize feet constraints ==
  wrench_leftFoot : Inport
  wrench_rightFoot : Inport  Port=2
  feetConstraints : Inport  Port=3
  state : Inport  Port=4
  Enable : EnablePort
  Feet Constraints : Scope  NumInputPorts=4
      settings: TimeRange=auto  ShowLegends=on  MaxDataPoints=5000  SaveToWorkspace=off  YMin=-53.15397~-98.95923~-0.125~-0.25  YMax=338.39155~343.38262~1.125~12.25  SampleTime=-1
  wires:
  state/1 -> Feet Constraints/4
  feetConstraints/1 -> Feet Constraints/3  "feetConstraints"
  wrench_rightFoot/1 -> Feet Constraints/2  "wrench_rightFoot"
  wrench_leftFoot/1 -> Feet Constraints/1  "wrench_leftFoot"

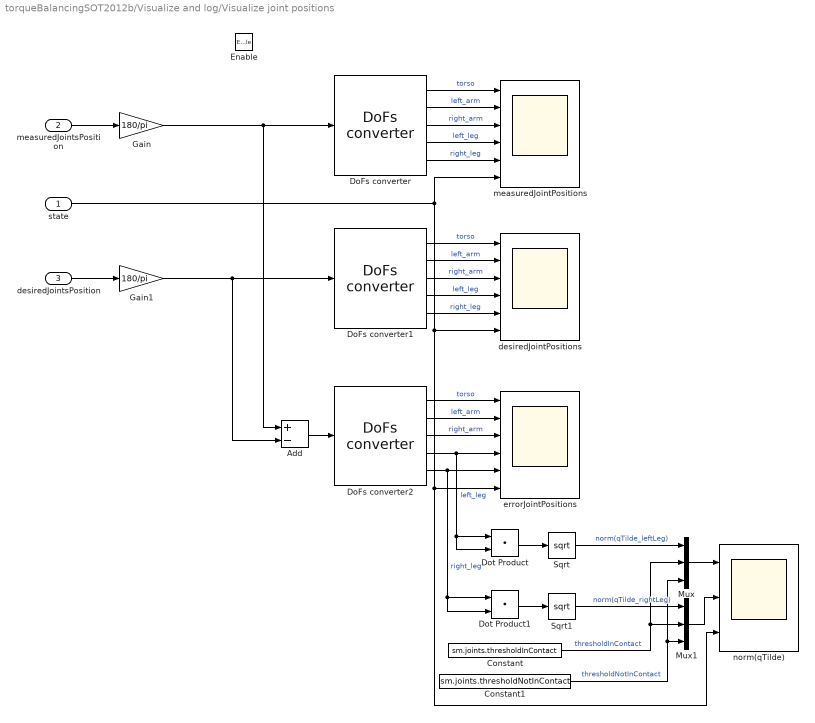
== system torqueBalancingSOT2012b/Visualize and log/Visualize joint positions ==
  state : Inport
  measuredJointsPosition : Inport  Port=2
  desiredJointsPosition : Inport  Port=3
  Enable : EnablePort
  Add : Sum  Inputs=+-
  Constant : Constant  Value=sm.joints.thresholdInContact
  Constant1 : Constant  Value=sm.joints.thresholdNotInContact
  DoFs converter : WBToolboxLibrary/Utilities/DoFs converter  yarp2WBIOption=From WBI to YARP  robotName=WBT_robotName  localName=WBT_modelName  wbiFile=WBT_wbiFilename  wbiList=WBT_wbiList
  DoFs converter1 : WBToolboxLibrary/Utilities/DoFs converter  yarp2WBIOption=From WBI to YARP  robotName=WBT_robotName  localName=WBT_modelName  wbiFile=WBT_wbiFilename  wbiList=WBT_wbiList
  DoFs converter2 : WBToolboxLibrary/Utilities/DoFs converter  yarp2WBIOption=From WBI to YARP  robotName=WBT_robotName  localName=WBT_modelName  wbiFile=WBT_wbiFilename  wbiList=WBT_wbiList
  Dot Product : DotProduct  InputSameDT=on  OutDataTypeStr=Inherit: Inherit via internal rule
  Dot Product1 : DotProduct  InputSameDT=on  OutDataTypeStr=Inherit: Inherit via internal rule
  Gain : Gain  Gain=180/pi
  Gain1 : Gain  Gain=180/pi
  Mux : Mux  Inputs=3
  Mux1 : Mux  Inputs=3
  Sqrt : Sqrt  SaturateOnIntegerOverflow=on
  Sqrt1 : Sqrt  SaturateOnIntegerOverflow=on
  desiredJointPositions : Scope  NumInputPorts=6
      settings: TimeRange=auto  ShowLegends=on  MaxDataPoints=5000  SaveName=desiredJointPositions  YMin=-10~-5~-5~-30~-30~0  YMax=10~5~5~30~30~12  SampleTime=-1  DataFormat=Structure  Decimation=2
  errorJointPositions : Scope  NumInputPorts=6
      settings: TimeRange=auto  ShowLegends=on  MaxDataPoints=5000  SaveName=errorJointPositions  YMin=-10~-5~-5~-30~-30~0  YMax=10~5~5~30~30~12  SampleTime=-1  DataFormat=Structure  Decimation=2
  measuredJointPositions : Scope  NumInputPorts=6
      settings: TimeRange=auto  ShowLegends=on  MaxDataPoints=5000  SaveName=measuredJointPositions  YMin=-10~-5~-5~-30~-30~0  YMax=10~5~5~30~30~12  SampleTime=-1  DataFormat=Structure  Decimation=2
  norm(qTilde) : Scope  NumInputPorts=3
      settings: TimeRange=auto  ShowLegends=on  MaxDataPoints=5000  YMin=-6.25~-6.25~-0.25  YMax=56.25~56.25~12.25  SampleTime=-1  DataFormat=Structure  Decimation=2
  wires:
  DoFs converter/5 -> measuredJointPositions/5  "right_leg"
  DoFs converter/4 -> measuredJointPositions/4  "left_leg"
  DoFs converter/2 -> measuredJointPositions/2  "left_arm"
  DoFs converter/1 -> measuredJointPositions/1  "torso"
  DoFs converter2/2 -> errorJointPositions/2  "left_arm"
  Gain1/1 -> Add/2, DoFs converter1/1
  DoFs converter2/1 -> errorJointPositions/1  "torso"
  desiredJointsPosition/1 -> Gain1/1
  measuredJointsPosition/1 -> Gain/1
  DoFs converter2/4 -> errorJointPositions/4, Dot Product/1, Dot Product/2  "left_leg"
  DoFs converter1/1 -> desiredJointPositions/1  "torso"
  DoFs converter1/3 -> desiredJointPositions/3  "right_arm"
  DoFs converter1/4 -> desiredJointPositions/4  "left_leg"
  Add/1 -> DoFs converter2/1
  Gain/1 -> Add/1, DoFs converter/1
  DoFs converter/3 -> measuredJointPositions/3  "right_arm"
  DoFs converter1/2 -> desiredJointPositions/2  "left_arm"
  DoFs converter2/3 -> errorJointPositions/3  "right_arm"
  DoFs converter2/5 -> errorJointPositions/5, Dot Product1/2, Dot Product1/1  "right_leg"
  DoFs converter1/5 -> desiredJointPositions/5  "right_leg"
  state/1 -> norm(qTilde)/3, errorJointPositions/6, desiredJointPositions/6, measuredJointPositions/6
  Dot Product/1 -> Sqrt/1
  Dot Product1/1 -> Sqrt1/1
  Sqrt/1 -> Mux/1  "norm(qTilde_leftLeg)"
  Sqrt1/1 -> Mux1/1  "norm(qTilde_rightLeg)"
  Constant/1 -> Mux/2, Mux1/2  "thresholdInContact"
  Constant1/1 -> Mux1/3, Mux/3  "thresholdNotInContact"
  Mux/1 -> norm(qTilde)/1
  Mux1/1 -> norm(qTilde)/2

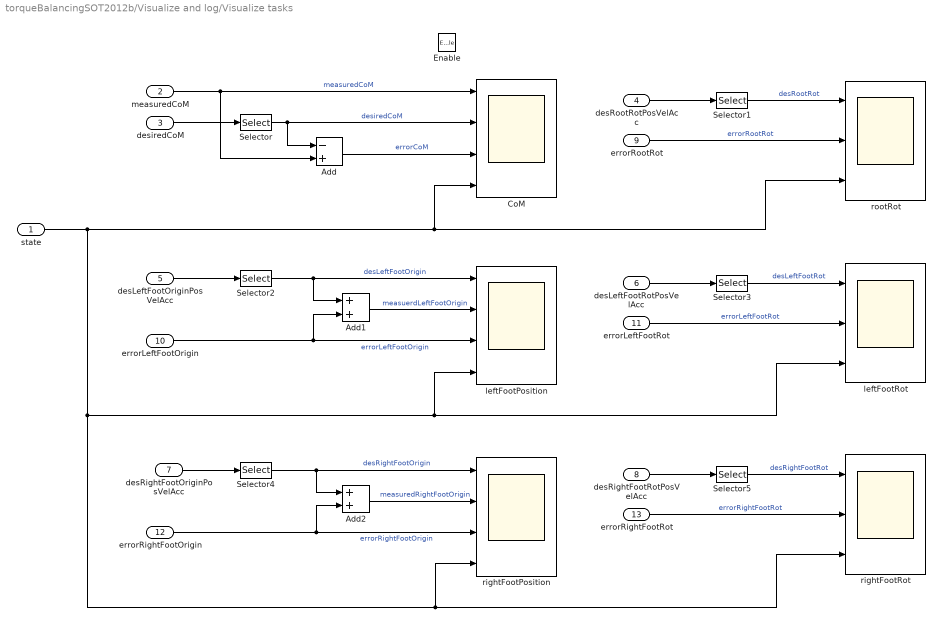
== system torqueBalancingSOT2012b/Visualize and log/Visualize tasks ==
  state : Inport
  measuredCoM : Inport  Port=2
  desiredCoM : Inport  Port=3
  desRootRotPosVelAcc : Inport  Port=4
  desLeftFootOriginPosVelAcc : Inport  Port=5
  desLeftFootRotPosVelAcc : Inport  Port=6
  desRightFootOriginPosVelAcc : Inport  Port=7
  desRightFootRotPosVelAcc : Inport  Port=8
  errorRootRot : Inport  Port=9
  errorLeftFootOrigin : Inport  Port=10
  errorLeftFootRot : Inport  Port=11
  errorRightFootOrigin : Inport  Port=12
  errorRightFootRot : Inport  Port=13
  Enable : EnablePort
  Add : Sum  Inputs=-+
  Add1 : Sum
  Add2 : Sum
  CoM : Scope  NumInputPorts=4
      settings: TimeRange=auto  ShowLegends=on  MaxDataPoints=5000  SaveName=CoM  YMin=-0.14117~-0.1407~-0.00736~0.375  YMax=0.58918~0.58526~0.01217~6.625  SampleTime=-1  DataFormat=Structure  Decimation=2
  Selector{,1..5} (6 alike) : Selector  NumberOfDimensions=2  InputPortWidth=9  IndexOptions=Index vector (dialog),Index vector (dialog)  Indices=[1:3],1  OutputSizes=1,1
  leftFootPosition : Scope  NumInputPorts=4
      settings: TimeRange=auto  ShowLegends=on  MaxDataPoints=5000  SaveName=leftFootPosition  YMin=-1.00000~-0.00000000000000044~-0.00000000000000044~0.375  YMax=1.00000~0.00000000000000038~0.00000000000000038~6.625  SampleTime=-1  DataFormat=Structure  Decimation=2
  leftFootRot : Scope  NumInputPorts=3
      settings: TimeRange=auto  ShowLegends=on  MaxDataPoints=5000  SaveName=leftFootRot  YMin=-0.125~-0.00000000000000017~0.375  YMax=1.125~0.00000000000000023~6.625  SampleTime=-1  DataFormat=Structure  Decimation=2
  rightFootPosition : Scope  NumInputPorts=4
      settings: TimeRange=auto  ShowLegends=on  MaxDataPoints=5000  SaveName=rightFootPosition  YMin=-0.15941~-0.16685~-0.02783~0.375  YMax=0.07318~0.05475~0.01468~6.625  SampleTime=-1  DataFormat=Structure  Decimation=2
  rightFootRot : Scope  NumInputPorts=3
      settings: TimeRange=auto  ShowLegends=on  MaxDataPoints=5000  SaveName=rightFootRot  YMin=-0.125~-0.02051~0.375  YMax=1.125~0.04273~6.625  SampleTime=-1  DataFormat=Structure  Decimation=2
  rootRot : Scope  NumInputPorts=3
      settings: TimeRange=auto  ShowLegends=on  MaxDataPoints=5000  SaveName=rootRot  YMin=-1.12582~-0.01374~0.375  YMax=0.13262~0.11922~6.625  SampleTime=-1  DataFormat=Structure  Decimation=2
  wires:
  Selector/1 -> Add/1, CoM/2  "desiredCoM"
  Add/1 -> CoM/3  "errorCoM"
  desiredCoM/1 -> Selector/1
  state/1 -> rootRot/3, CoM/4, rightFootRot/3, rightFootPosition/4, leftFootPosition/4, leftFootRot/3
  measuredCoM/1 -> Add/2, CoM/1  "measuredCoM"
  Selector1/1 -> rootRot/1  "desRootRot"
  desLeftFootOriginPosVelAcc/1 -> Selector2/1
  desLeftFootRotPosVelAcc/1 -> Selector3/1
  desRightFootOriginPosVelAcc/1 -> Selector4/1
  desRightFootRotPosVelAcc/1 -> Selector5/1
  errorRootRot/1 -> rootRot/2  "errorRootRot"
  errorLeftFootRot/1 -> leftFootRot/2  "errorLeftFootRot"
  errorLeftFootOrigin/1 -> Add1/2, leftFootPosition/3  "errorLeftFootOrigin"
  errorRightFootOrigin/1 -> Add2/2, rightFootPosition/3  "errorRightFootOrigin"
  errorRightFootRot/1 -> rightFootRot/2  "errorRightFootRot"
  desRootRotPosVelAcc/1 -> Selector1/1
  Selector2/1 -> Add1/1, leftFootPosition/1  "desLeftFootOrigin"
  Add1/1 -> leftFootPosition/2  "measuerdLeftFootOrigin"
  Selector3/1 -> leftFootRot/1  "desLeftFootRot"
  Selector4/1 -> Add2/1, rightFootPosition/1  "desRightFootOrigin"
  Add2/1 -> rightFootPosition/2  "measuredRightFootOrigin"
  Selector5/1 -> rightFootRot/1  "desRightFootRot"

== system torqueBalancingSOT2012b/Visualize and log/Visualize torques ==
  state : Inport
  measuredJointsTorque : Inport  Port=2
  desiredJointsTorque : Inport  Port=3
  Enable : EnablePort
  Add : Sum  Inputs=+-
  DoFs converter : WBToolboxLibrary/Utilities/DoFs converter  yarp2WBIOption=From WBI to YARP  robotName=WBT_robotName  localName=WBT_modelName  wbiFile=WBT_wbiFilename  wbiList=WBT_wbiList
  DoFs converter1 : WBToolboxLibrary/Utilities/DoFs converter  yarp2WBIOption=From WBI to YARP  robotName=WBT_robotName  localName=WBT_modelName  wbiFile=WBT_wbiFilename  wbiList=WBT_wbiList
  DoFs converter2 : WBToolboxLibrary/Utilities/DoFs converter  yarp2WBIOption=From WBI to YARP  robotName=WBT_robotName  localName=WBT_modelName  wbiFile=WBT_wbiFilename  wbiList=WBT_wbiList
  desiredJointTorques : Scope  NumInputPorts=6
      settings: TimeRange=auto  ShowLegends=on  MaxDataPoints=5000  SaveName=desiredJointTorques  YMin=-10~-5~-5~-30~-30~0  YMax=10~5~5~30~30~12  SampleTime=-1  DataFormat=Structure  Decimation=2
  errorJointTorques : Scope  NumInputPorts=6
      settings: TimeRange=auto  ShowLegends=on  MaxDataPoints=5000  SaveName=errorJointTorques  YMin=-10~-5~-5~-30~-30~0  YMax=10~5~5~30~30~12  SampleTime=-1  DataFormat=Structure  Decimation=2
  measuredJointTorques : Scope  NumInputPorts=6
      settings: TimeRange=auto  ShowLegends=on  MaxDataPoints=5000  SaveName=measuredJointTorques  YMin=-10~-5~-5~-30~-30~0  YMax=10~5~5~30~30~12  SampleTime=-1  DataFormat=Structure  Decimation=2
  wires:
  DoFs converter1/2 -> desiredJointTorques/2  "left_arm"
  DoFs converter2/3 -> errorJointTorques/3  "right_arm"
  DoFs converter2/5 -> errorJointTorques/5  "right_leg"
  DoFs converter2/1 -> errorJointTorques/1  "torso"
  DoFs converter/5 -> measuredJointTorques/5  "right_leg"
  DoFs converter/4 -> measuredJointTorques/4  "left_leg"
  DoFs converter/2 -> measuredJointTorques/2  "left_arm"
  DoFs converter/1 -> measuredJointTorques/1  "torso"
  desiredJointsTorque/1 -> DoFs converter1/1, Add/2
  measuredJointsTorque/1 -> Add/1, DoFs converter/1
  DoFs converter/3 -> measuredJointTorques/3  "right_arm"
  DoFs converter2/4 -> errorJointTorques/4  "left_leg"
  DoFs converter1/1 -> desiredJointTorques/1  "torso"
  DoFs converter1/3 -> desiredJointTorques/3  "right_arm"
  DoFs converter1/4 -> desiredJointTorques/4  "left_leg"
  DoFs converter2/2 -> errorJointTorques/2  "left_arm"
  Add/1 -> DoFs converter2/1
  DoFs converter1/5 -> desiredJointTorques/5  "right_leg"
  state/1 -> measuredJointTorques/6, errorJointTorques/6, desiredJointTorques/6

== system torqueBalancingSOT2012b/synchronizer/GAZEBO_SYNCHRONIZER ==
  Enable : EnablePort
  Simulator Synchronizer : WBToolboxLibrary/Utilities/Simulator Synchronizer  period=CONFIG.Ts  serverPortName='/clock/rpc'  clientPortName='/WBT_synchronizer/rpc:o'

== system torqueBalancingSOT2012b/synchronizer/REAL_TIME_SYNC ==
  Enable : EnablePort
  Real Time Synchronizer : WBToolboxLibrary/Utilities/Real Time Synchronizer  period=CONFIG.Ts

== system torqueBalancingSOT2012b/Desired values/State Machine Walking/nu (vb + dqj) ==
  qj : Inport
  dqj : Inport  Port=2
  w_H_b : Inport  Port=3
  feetConstraints : Inport  Port=4
  Jacobian : WBToolboxLibrary/wholeBodyModel/Jacobians/Jacobian  frameName='l_sole'  robotName=WBT_robotName  localName=WBT_modelName  wbiFile=WBT_wbiFilename  wbiList=WBT_wbiList
  Jacobian1 : WBToolboxLibrary/wholeBodyModel/Jacobians/Jacobian  frameName='r_sole'  robotName=WBT_robotName  localName=WBT_modelName  wbiFile=WBT_wbiFilename  wbiList=WBT_wbiList
  Mux2 : Mux  Inputs=2
  baseVelocityFCN : MATLAB Function  TreatAsAtomicUnit=on
      settings: PermitHierarchicalResolution=ParametersOnly
  nu : Outport
  wires:
  qj/1 -> Jacobian1/2, Jacobian/2
  Jacobian1/1 -> baseVelocityFCN/2(JcRightFoot)
  dqj/1 -> Mux2/2, baseVelocityFCN/4(dqj)
  baseVelocityFCN/1(vb) -> Mux2/1
  w_H_b/1 -> Jacobian/1, Jacobian1/1
  feetConstraints/1 -> baseVelocityFCN/3(feetConstraints)
  Jacobian/1 -> baseVelocityFCN/1(JcLeftFoot)
  Mux2/1 -> nu/1

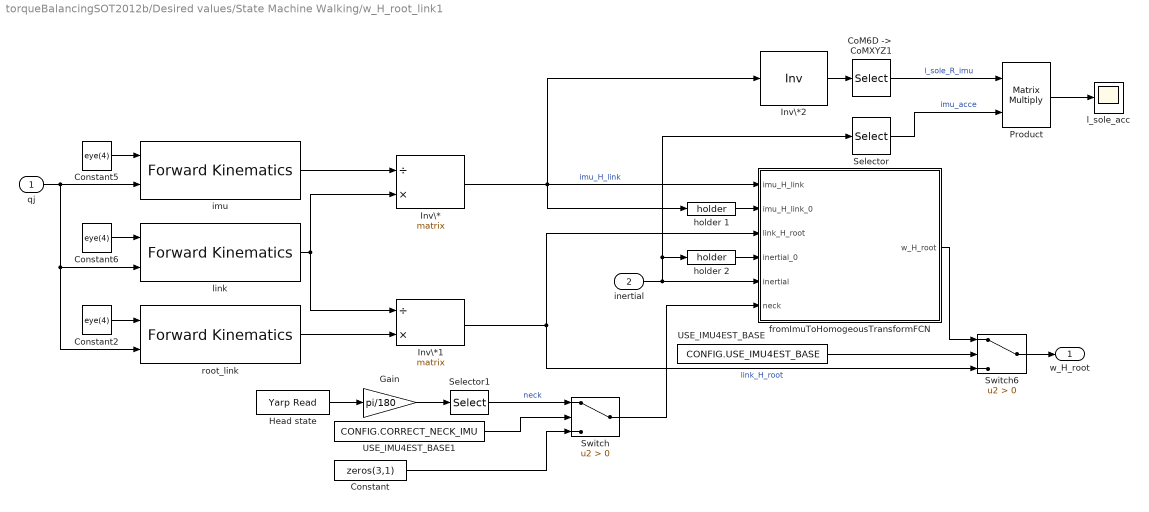
== system torqueBalancingSOT2012b/Desired values/State Machine Walking/w_H_root_link1 ==
  qj : Inport
  inertial : Inport  Port=2
  "CoM6D ->  CoMXYZ1" : Selector  NumberOfDimensions=2  InputPortWidth=7  IndexOptions=Index vector (dialog),Index vector (dialog)  Indices=[1 2 3],[1 2 3]  OutputSizes=1,1
  Constant : Constant  Value=zeros(3,1)
  Constant2 : Constant  Value=eye(4)
  Constant5 : Constant  Value=eye(4)
  Constant6 : Constant  Value=eye(4)
  Gain : Gain  Gain=pi/180
  Head state : WBToolboxLibrary/Utilities/Yarp Read  portName=[WBT_robotName, '/head/state:o']  signalSize=6  blocking=off  timestamp=off  autoconnect=on  errorOnConnection=off
  Inv\* : Product  Inputs=/*  Multiplication=Matrix(*)
  Inv\*1 : Product  Inputs=/*  Multiplication=Matrix(*)
  Inv\*2 : Product  Inputs=/  Multiplication=Matrix(*)
  Product : Product  Multiplication=Matrix(*)
  Selector : Selector  InputPortWidth=12  IndexOptions=Index vector (dialog)  Indices=[4 5 6 ]  OutputSizes=1
  Selector1 : Selector  InputPortWidth=6  IndexOptions=Index vector (dialog)  Indices=[1:3]  OutputSizes=1
  Switch : Switch  Criteria=u2 > Threshold
  Switch6 : Switch  Criteria=u2 > Threshold
  USE_IMU4EST_BASE : Constant  Value=CONFIG.USE_IMU4EST_BASE
  USE_IMU4EST_BASE1 : Constant  Value=CONFIG.CORRECT_NECK_IMU
  fromImuToHomogeousTransformFCN : MATLAB Function  TreatAsAtomicUnit=on
      settings: PermitHierarchicalResolution=ParametersOnly
  holder 1 : WBToolboxLibrary/Utilities/holder 
  holder 2 : WBToolboxLibrary/Utilities/holder 
  imu : WBToolboxLibrary/wholeBodyModel/Kinematics/Forward Kinematics  frameName='imu_frame'  robotName=WBT_robotName  localName=WBT_modelName  wbiFile=WBT_wbiFilename  wbiList=WBT_wbiList
  l_sole_acc : Scope
      settings: TimeRange=60  ShowLegends=on  MaxDataPoints=5000  SaveToWorkspace=off  YMin=-4.47309  YMax=14.2668  SampleTime=-1
  link : WBToolboxLibrary/wholeBodyModel/Kinematics/Forward Kinematics  frameName=link_name  robotName=WBT_robotName  localName=WBT_modelName  wbiFile=WBT_wbiFilename  wbiList=WBT_wbiList
  root_link : WBToolboxLibrary/wholeBodyModel/Kinematics/Forward Kinematics  frameName='root_link'  robotName=WBT_robotName  localName=WBT_modelName  wbiFile=WBT_wbiFilename  wbiList=WBT_wbiList
  w_H_root : Outport
  wires:
  Constant5/1 -> imu/1
  Inv\*/1 -> Inv\*2/1, holder 1/1, fromImuToHomogeousTransformFCN/1(imu_H_link)  "imu_H_link"
  imu/1 -> Inv\*/1
  Constant6/1 -> link/1
  Inv\*1/1 -> Switch6/3, fromImuToHomogeousTransformFCN/3(link_H_root)  "link_H_root"
  link/1 -> Inv\*/2, Inv\*1/1
  inertial/1 -> Selector/1, holder 2/1, fromImuToHomogeousTransformFCN/5(inertial)
  Switch6/1 -> w_H_root/1
  USE_IMU4EST_BASE/1 -> Switch6/2
  fromImuToHomogeousTransformFCN/1(w_H_root) -> Switch6/1
  Constant2/1 -> root_link/1
  qj/1 -> root_link/2, link/2, imu/2
  root_link/1 -> Inv\*1/2
  holder 1/1 -> fromImuToHomogeousTransformFCN/2(imu_H_link_0)
  holder 2/1 -> fromImuToHomogeousTransformFCN/4(inertial_0)
  Inv\*2/1 -> "CoM6D ->  CoMXYZ1"/1
  "CoM6D ->  CoMXYZ1"/1 -> Product/1  "l_sole_R_imu"
  Selector/1 -> Product/2  "imu_acce"
  Product/1 -> l_sole_acc/1
  Head state/1 -> Gain/1
  Selector1/1 -> Switch/1  "neck"
  USE_IMU4EST_BASE1/1 -> Switch/2
  Switch/1 -> fromImuToHomogeousTransformFCN/6(neck)
  Gain/1 -> Selector1/1
  Constant/1 -> Switch/3

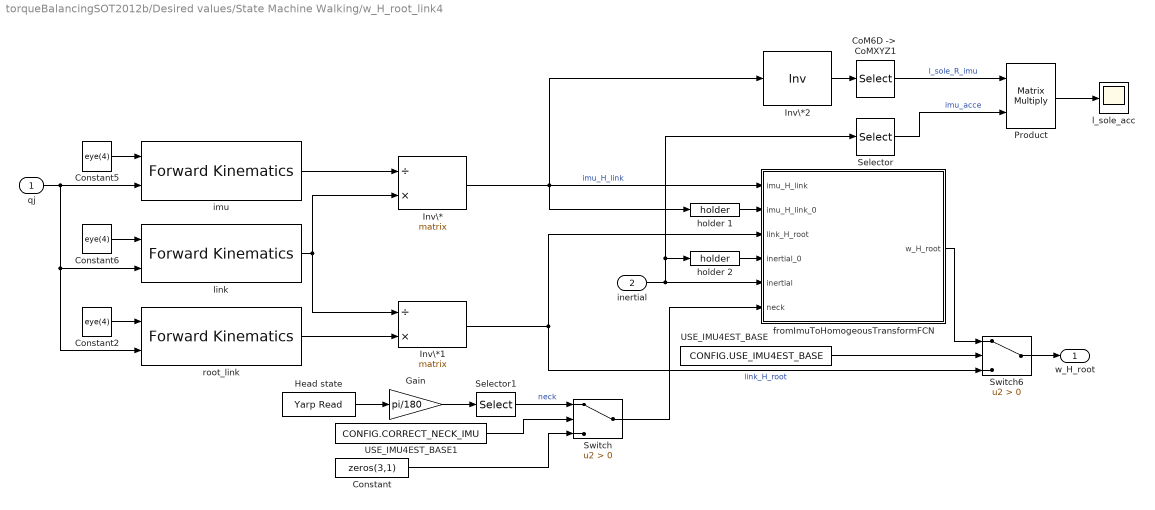
== system torqueBalancingSOT2012b/Desired values/State Machine Walking/w_H_root_link4 ==
  qj : Inport
  inertial : Inport  Port=2
  "CoM6D ->  CoMXYZ1" : Selector  NumberOfDimensions=2  InputPortWidth=7  IndexOptions=Index vector (dialog),Index vector (dialog)  Indices=[1 2 3],[1 2 3]  OutputSizes=1,1
  Constant : Constant  Value=zeros(3,1)
  Constant2 : Constant  Value=eye(4)
  Constant5 : Constant  Value=eye(4)
  Constant6 : Constant  Value=eye(4)
  Gain : Gain  Gain=pi/180
  Head state : WBToolboxLibrary/Utilities/Yarp Read  portName=[WBT_robotName, '/head/state:o']  signalSize=6  blocking=off  timestamp=off  autoconnect=on  errorOnConnection=off
  Inv\* : Product  Inputs=/*  Multiplication=Matrix(*)
  Inv\*1 : Product  Inputs=/*  Multiplication=Matrix(*)
  Inv\*2 : Product  Inputs=/  Multiplication=Matrix(*)
  Product : Product  Multiplication=Matrix(*)
  Selector : Selector  InputPortWidth=12  IndexOptions=Index vector (dialog)  Indices=[4 5 6 ]  OutputSizes=1
  Selector1 : Selector  InputPortWidth=6  IndexOptions=Index vector (dialog)  Indices=[1:3]  OutputSizes=1
  Switch : Switch  Criteria=u2 > Threshold
  Switch6 : Switch  Criteria=u2 > Threshold
  USE_IMU4EST_BASE : Constant  Value=CONFIG.USE_IMU4EST_BASE
  USE_IMU4EST_BASE1 : Constant  Value=CONFIG.CORRECT_NECK_IMU
  fromImuToHomogeousTransformFCN : MATLAB Function  TreatAsAtomicUnit=on
      settings: PermitHierarchicalResolution=ParametersOnly
  holder 1 : WBToolboxLibrary/Utilities/holder 
  holder 2 : WBToolboxLibrary/Utilities/holder 
  imu : WBToolboxLibrary/wholeBodyModel/Kinematics/Forward Kinematics  frameName='imu_frame'  robotName=WBT_robotName  localName=WBT_modelName  wbiFile=WBT_wbiFilename  wbiList=WBT_wbiList
  l_sole_acc : Scope
      settings: TimeRange=60  ShowLegends=on  MaxDataPoints=5000  SaveToWorkspace=off  YMin=-4.47309  YMax=14.2668  SampleTime=-1
  link : WBToolboxLibrary/wholeBodyModel/Kinematics/Forward Kinematics  frameName=link_name  robotName=WBT_robotName  localName=WBT_modelName  wbiFile=WBT_wbiFilename  wbiList=WBT_wbiList
  root_link : WBToolboxLibrary/wholeBodyModel/Kinematics/Forward Kinematics  frameName='root_link'  robotName=WBT_robotName  localName=WBT_modelName  wbiFile=WBT_wbiFilename  wbiList=WBT_wbiList
  w_H_root : Outport
  wires:
  Constant5/1 -> imu/1
  Inv\*/1 -> Inv\*2/1, holder 1/1, fromImuToHomogeousTransformFCN/1(imu_H_link)  "imu_H_link"
  imu/1 -> Inv\*/1
  Constant6/1 -> link/1
  Inv\*1/1 -> Switch6/3, fromImuToHomogeousTransformFCN/3(link_H_root)  "link_H_root"
  link/1 -> Inv\*/2, Inv\*1/1
  inertial/1 -> Selector/1, holder 2/1, fromImuToHomogeousTransformFCN/5(inertial)
  Switch6/1 -> w_H_root/1
  USE_IMU4EST_BASE/1 -> Switch6/2
  fromImuToHomogeousTransformFCN/1(w_H_root) -> Switch6/1
  Constant2/1 -> root_link/1
  qj/1 -> root_link/2, link/2, imu/2
  root_link/1 -> Inv\*1/2
  holder 1/1 -> fromImuToHomogeousTransformFCN/2(imu_H_link_0)
  holder 2/1 -> fromImuToHomogeousTransformFCN/4(inertial_0)
  Inv\*2/1 -> "CoM6D ->  CoMXYZ1"/1
  "CoM6D ->  CoMXYZ1"/1 -> Product/1  "l_sole_R_imu"
  Selector/1 -> Product/2  "imu_acce"
  Product/1 -> l_sole_acc/1
  Head state/1 -> Gain/1
  Selector1/1 -> Switch/1  "neck"
  USE_IMU4EST_BASE1/1 -> Switch/2
  Switch/1 -> fromImuToHomogeousTransformFCN/6(neck)
  Gain/1 -> Selector1/1
  Constant/1 -> Switch/3
